simulink library "lib_Convection_LamCircTurbAnnulus"  (R2015a)
settings: Solver=ode45  StartTime=0.0  StopTime=10.0  RelTol=1e-3
settings Model: Creator=jlkratz  LastModifiedBy=jlkratz

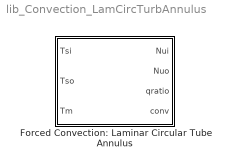
== system lib_Convection_LamCircTurbAnnulus ==
  Forced Convection: Laminar Circular Tube Annulus : Subsystem  mask(TSAT: Forced Convection: Laminar Circular Tube Annulus){Scenario_M=Both surfaces maintain a uniform heat flux, DioDo_M=[0.01 0.5], BN_M=double(gcb)}
      mask prompts: Scenario_M "Scenario_M - Heat transfer scenario"; DioDo_M "DioDo_M - Ratio of inner tube diamter to outer tube diameter (Di/Do) - value(s) shoud be between 0 and 1, if they are not they will be truncated to this range."; BN_M "BN_M - Block Name"
      mask help:
      | This block provides the Nusselt number for fully developed laminar flow within a circular annulus tube. There are two options:
      |
      | (1) one side is insulated and the other has a constant temperature
      | (2) uniform heat flux is maintained at both surfaces
      |
      | The block outputs are the Nusselt numbers associated with the inner and outer surfaces. In case (2) the solutions involves an iterative solver whose solution (the ratio of heat flux's qi/qo) and a parameter indicating convergence of the solution is output. This case also requires additional inputs which include the temperature of both surfaces and the mean temperature of the fluid. Note that the hydraulic diameter, Do - Di in this case, should be used to calculate the convective heat transfer coefficient using the Nusselt numbers from this block.
      |
      | For turbulent flows a circular tube correlation, such as the Dittus-Boelter equation, can be used to get a first approximation of the Nusselt number for both surfaces assuming they are equal and the hydraulic diameter should be used. For more information about this block see the block help menu.
      mask init:
      | %Setup Inputs ------------------------------------------------------------%
      | 
      | % Inport Numbers
      | n = 1; %first inport number
      | 
      | % Inner Surface Temperature (Tsi)
      | if Scenario_M == 2
      |     if strcmp(get_param([gcb '/Tsi'],'BlockType'),'Constant')
      |         MSK_ReplaceBlock_TMATS([gcb '/Tsi'],'built-in/Inport');
      |     end
      |     set_param([gcb '/Tsi'],'Port',num2str(n));
      |     n = n + 1;
      | else
      |     if strcmp(get_param([gcb '/Tsi'],'BlockType'),'Inport')
      |         MSK_ReplaceBlock_TMATS([gcb '/Tsi'],'built-in/Constant');
      |         set_param([gcb '/Tsi'],'Value','700');
      |     end
      | end
      | 
      | % Outer Surface Temperature (Tso)
      | if Scenario_M == 2
      |     if strcmp(get_param([gcb '/Tso'],'BlockType'),'Constant')
      |         MSK_ReplaceBlock_TMATS([gcb '/Tso'],'built-in/Inport');
      |     end
      |     set_param([gcb '/Tso'],'Port',num2str(n));
      |     n = n + 1;
      | else
      |     if strcmp(get_param([gcb '/Tso'],'BlockType'),'Inport')
      |         MSK_ReplaceBlock_TMATS([gcb '/Tso'],'built-in/Constant');
      |         set_param([gcb '/Tso'],'Value','500');
      |     end
      | end
      | 
      | % Mean Fluid Temperature (Tm)
      | if Scenario_M == 2
      |     if strcmp(get_param([gcb '/Tm'],'BlockType'),'Constant')
      |         MSK_ReplaceBlock_TMATS([gcb '/Tm'],'built-in/Inport');
      |     end
      |     set_param([gcb '/Tm'],'Port',num2str(n));
      |     n = n + 1;
      | else
      |     if strcmp(get_param([gcb '/Tm'],'BlockType'),'Inport')
      |         MSK_ReplaceBlock_TMATS([gcb '/Tm'],'built-in/Constant');
      |         set_param([gcb '/Tm'],'Value','400');
      |     end
      | end
      | 
      | %Setup Outputs -----------------------------------------------------------%
      | 
      | % Outport Numbers
      | n = 3; %first inport number
      | 
      | % Uniform heat flux ratio (qratio)
      | if Scenario_M == 2
      |     if strcmp(get_param([gcb '/qratio'],'BlockType'),'Terminator')
      |         MSK_ReplaceBlock_TMATS([gcb '/qratio'],'built-in/Outport');
      |     end
      |     set_param([gcb '/qratio'],'Port',num2str(n));
      |     n = n + 1;
      | else
      |     if strcmp(get_param([gcb '/qratio'],'BlockType'),'Outport')
      |         MSK_ReplaceBlock_TMATS([gcb '/qratio'],'built-in/Terminator');
      |         %set_param([gcb '/qratio'],'Value','1');
      |     end
      | end
      | 
      | % Convergence varialbe for qratio solution (conv)
      | if Scenario_M == 2
      |     if strcmp(get_param([gcb '/conv'],'BlockType'),'Terminator')
      |         MSK_ReplaceBlock_TMATS([gcb '/conv'],'built-in/Outport');
      |     end
      |     set_param([gcb '/conv'],'Port',num2str(n));
      |     n = n + 1;
      | else
      |     if strcmp(get_param([gcb '/conv'],'BlockType'),'Outport')
      |         MSK_ReplaceBlock_TMATS([gcb '/conv'],'built-in/Terminator');
      |         %set_param([gcb '/conv'],'Value','1');
      |     end
      | end
      mask Help: web(which('Convection_TSAT_LamCircTubeAnnulus.html'),'-helpbrowser')
      mask TypeOptions Scenario_M: One surface is insulated and the other is at a constant temperature | Both surfaces maintain a uniform heat flux

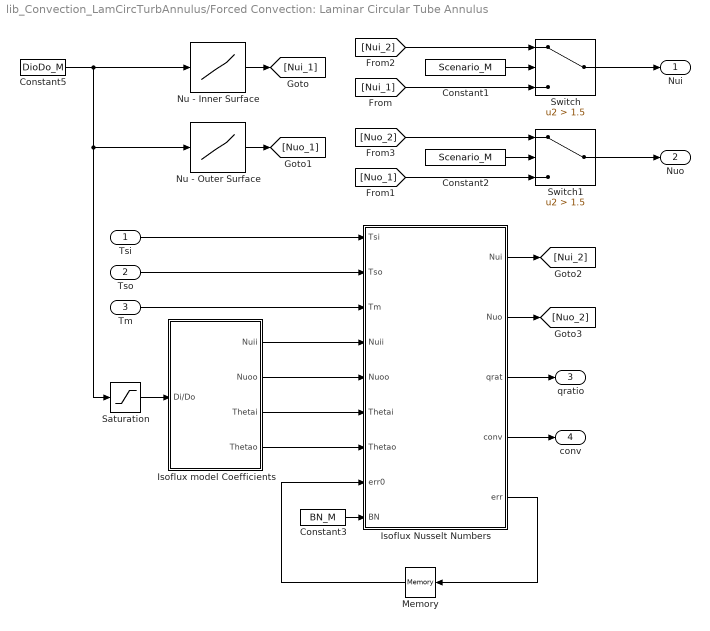
== system lib_Convection_LamCircTurbAnnulus/Forced Convection: Laminar Circular Tube Annulus ==
  Tsi : Inport
  Tso : Inport  Port=2
  Tm : Inport  Port=3
  Constant1 : Constant  Value=Scenario_M
  Constant2 : Constant  Value=Scenario_M
  Constant3 : Constant  Value=BN_M
  Constant5 : Constant  Value=DioDo_M
  Isoflux Nusselt Numbers : MATLAB Function  TreatAsAtomicUnit=on
  "Isoflux model Coefficients " : Subsystem
  Memory : Memory  X0=zeros(1,10)
  Nu - Inner Surface : Lookup_n-D  NumberOfTableDimensions=1  BreakpointsForDimension1=[0 0.05 0.1 0.25 0.5 1]  Table=[17.46 17.46 11.56 7.37 5.74 4.86]  InternalRulePriority=Speed  RndMeth=Simplest  InputSameDT=on
  Nu - Outer Surface : Lookup_n-D  NumberOfTableDimensions=1  BreakpointsForDimension1=[0 0.05 0.1 0.25 0.5 1]  Table=[3.66 4.06 4.11 4.23 4.43 4.86]  InternalRulePriority=Speed  RndMeth=Simplest  InputSameDT=on
  Saturation : Saturate  UpperLimit=1  LowerLimit=0.000001
  Switch : Switch  Criteria=u2 > Threshold  Threshold=1.5
  Switch1 : Switch  Criteria=u2 > Threshold  Threshold=1.5
  Nui : Outport
  Nuo : Outport  Port=2
  qratio : Outport  Port=3
  conv : Outport  Port=4
  wires:
  Saturation/1 -> "Isoflux model Coefficients "/1(Di/Do)
  Memory/1 -> Isoflux Nusselt Numbers/8(err0)
  Constant3/1 -> Isoflux Nusselt Numbers/9(BN)
  Isoflux Nusselt Numbers/5(err) -> Memory/1
  Switch1/1 -> Nuo/1
  Switch/1 -> Nui/1
  Constant2/1 -> Switch1/2
  [Nuo_1] -> Switch1/3
  [Nuo_2] -> Switch1/1
  [Nui_1] -> Switch/3
  [Nui_2] -> Switch/1
  Constant1/1 -> Switch/2
  "Isoflux model Coefficients "/4(Thetao) -> Isoflux Nusselt Numbers/7(Thetao)
  "Isoflux model Coefficients "/3(Thetai) -> Isoflux Nusselt Numbers/6(Thetai)
  "Isoflux model Coefficients "/2(Nuoo) -> Isoflux Nusselt Numbers/5(Nuoo)
  "Isoflux model Coefficients "/1(Nuii) -> Isoflux Nusselt Numbers/4(Nuii)
  Constant5/1 -> Nu - Outer Surface/1, Saturation/1, Nu - Inner Surface/1
  Tm/1 -> Isoflux Nusselt Numbers/3(Tm)
  Tso/1 -> Isoflux Nusselt Numbers/2(Tso)
  Tsi/1 -> Isoflux Nusselt Numbers/1(Tsi)
  Isoflux Nusselt Numbers/4(conv) -> conv/1
  Isoflux Nusselt Numbers/3(qrat) -> qratio/1
  Isoflux Nusselt Numbers/2(Nuo) -> [Nuo_2]
  Isoflux Nusselt Numbers/1(Nui) -> [Nui_2]
  Nu - Outer Surface/1 -> [Nuo_1]
  Nu - Inner Surface/1 -> [Nui_1]

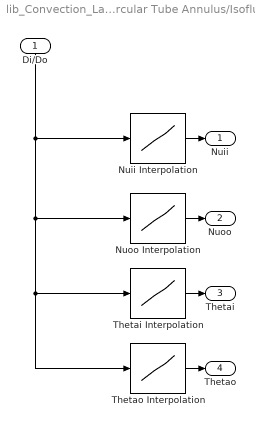
== system lib_Convection_LamCircTurbAnnulus/Forced Convection: Laminar Circular Tube Annulus/Isoflux model Coefficients  ==
  Di/Do : Inport
  Nuii Interpolation : Lookup_n-D  NumberOfTableDimensions=1  BreakpointsForDimension1=[0 0.000001 0.05 0.1 0.2 0.4 0.6 0.8 1]  Table=[0 17.81 17.81 11.91 8.499 6.583 5.912 5.58 5.385]  InternalRulePriority=Speed  RndMeth=Simplest  InputSameDT=on
  Nuoo Interpolation : Lookup_n-D  NumberOfTableDimensions=1  BreakpointsForDimension1=[0 0.05 0.1 0.2 0.4 0.6 0.8 1]  Table=[4.364 4.792 4.834 4.833 4.979 5.099 5.24 5.385]  InternalRulePriority=Speed  RndMeth=Simplest  InputSameDT=on
  Thetai Interpolation : Lookup_n-D  NumberOfTableDimensions=1  BreakpointsForDimension1=[0 0.000001 0.05 0.1 0.2 0.4 0.6 0.8 1]  Table=[0 2.18 2.18 1.383 0.905 0.603 0.473 0.401 0.346]  InternalRulePriority=Speed  RndMeth=Simplest  InputSameDT=on
  Thetao Interpolation : Lookup_n-D  NumberOfTableDimensions=1  BreakpointsForDimension1=[0 0.05 0.1 0.2 0.4 0.6 0.8 1]  Table=[0 0.0294 0.0562 0.1041 0.1823 0.2455 0.299 0.346]  InternalRulePriority=Speed  RndMeth=Simplest  InputSameDT=on
  Nuii : Outport
  Nuoo : Outport  Port=2
  Thetai : Outport  Port=3
  Thetao : Outport  Port=4
  wires:
  Nuii Interpolation/1 -> Nuii/1
  Nuoo Interpolation/1 -> Nuoo/1
  Thetao Interpolation/1 -> Thetao/1
  Di/Do/1 -> Nuii Interpolation/1, Nuoo Interpolation/1, Thetai Interpolation/1, Thetao Interpolation/1
  Thetai Interpolation/1 -> Thetai/1

== matlab function lib_Convection_LamCircTurbAnnulus/Forced Convection: Laminar Circular Tube Annulus/Isoflux Nusselt Numbers ==
  data: Nui output; Nuo output; qrat output; conv output; Tsi input; Tso input; Tm input; Nuii input; Nuoo input; Thetai input; Thetao input; err0 input; BN input; err output
function [Nui,Nuo,qrat,conv,err] = IsofluxSurfaces(Tsi, Tso, Tm, Nuii, Nuoo, Thetai, Thetao, err0, BN)
%#codegen

%Warning/Error Check
err = err0;
errNum = 1;
%Tsi is a 1-D array?
if min(size(Tsi)) ~= 1 && err0(errNum) ~= 1
    fprintf('warning in %s: Tsi must be a scalar or 1-D array\n',char(BN));
    err(errNum) = 1;
end
errNum = errNum + 1;
%Tso is a 1-D array?
if min(size(Tso)) ~= 1 && err0(errNum) ~= 1
    fprintf('warning in %s: Tso must be a scalar or 1-D array\n',char(BN));
    err(errNum) = 1;
end
errNum = errNum + 1;
%Tm is a 1-D array?
if min(size(Tm)) ~= 1 && err0(errNum) ~= 1
    fprintf('warning in %s: Tm must be a scalar or 1-D array\n',char(BN));
    err(errNum) = 1;
end
errNum = errNum + 1;
%Tsi, Tso, Tm, and DioDo_m (Nuii, Nuoo, Thetai, and Thetao) are the same size?
if (length(Tsi) ~= length(Tso) || length(Tsi) ~= length(Tm) || length(Tsi) ~= length(Nuii)) && err0(errNum) ~= 1
    fprintf('warning in %s: Tsi, Tso, Tm and DioDo_M must have the same number of elements\n',char(BN));
    err(errNum) = 1;
end
errNum = errNum + 1;
%Tsi has all real elements?
if min(isreal(Tsi)) < 1 && err0(errNum) ~= 1
    fprintf('warning in %s: Tsi must have all real elements\n',char(BN));
    err(errNum) = 1;
end
errNum = errNum + 1;
%Tso has all real elements?
if min(isreal(Tso)) < 1 && err0(errNum) ~= 1
    fprintf('warning in %s: Tso must have all real elements\n',char(BN));
    err(errNum) = 1;
end
errNum = errNum + 1;
%Tm has all real elements?
if min(isreal(Tm)) < 1 && err0(errNum) ~= 1
    fprintf('warning in %s: Tm must have all real elements\n',char(BN));
    err(errNum) = 1;
end
errNum = errNum + 1;
%Tsi has all finite elements?
if (max(isnan(Tsi)) > 0 || max(isinf(Tsi)) > 0) && err0(errNum) ~= 1
    fprintf('warning in %s: Tsi must have all finite elements\n',char(BN));
    err(errNum) = 1;
end
errNum = errNum + 1;
%Tso has all finite elements?
if (max(isnan(Tso)) > 0 || max(isinf(Tso)) > 0) && err0(errNum) ~= 1
    fprintf('warning in %s: Tso must have all finite elements\n',char(BN));
    err(errNum) = 1;
end
%Tm has all finite elements?
if (max(isnan(Tm)) > 0 || max(isinf(Tm)) > 0) && err0(errNum) ~= 1
    fprintf('warning in %s: Tm must have all finite elements\n',char(BN));
    err(errNum) = 1;
end

%Max number of iterations
imax = 1000;

%Initialize outputs
Nui = zeros(1,length(Tsi));
Nuo = zeros(1,length(Tsi));
qrat = zeros(1,length(Tsi));
conv = zeros(1,length(Tsi));

for j = 1:length(Tsi)

    %vector of the variable being solve for
    dT1 = Tsi(j) - Tm(j);
    dT2 = Tso(j) - Tm(j);
    a = abs(15*dT1/dT2);
    n = 100;
    qrat_vect = linspace(-a,a,n);

    %find the appropriate root
    if sign(Tsi(j)-Tm(j)) == sign(Tso(j)-Tm(j))
        Fend = qrat_vect(end) - (Nuii(j)/(1 - (1/qrat_vect(end))*Thetai(j))) * ((1 - qrat_vect(end)*Thetao(j))/Nuoo(j)) * (Tsi(j) - Tm(j))/(Tso(j) - Tm(j));
        signFend = sign(Fend);
        i = length(qrat_vect)-1;
        cnt = 0;
        Fi = qrat_vect(i) - (Nuii(j)/(1 - (1/qrat_vect(i))*Thetai(j))) * ((1 - qrat_vect(i)*Thetao(j))/Nuoo(j)) * (Tsi(j) - Tm(j))/(Tso(j) - Tm(j));
        while sign(Fi) == signFend && cnt < imax
            i = i - 1;
            cnt = cnt + 1;
            Fi = qrat_vect(i) - (Nuii(j)/(1 - (1/qrat_vect(i))*Thetai(j))) * ((1 - qrat_vect(i)*Thetao(j))/Nuoo(j)) * (Tsi(j) - Tm(j))/(Tso(j) - Tm(j));
        end
        conv(j) = 1;
        if cnt == imax
            conv(j) = 0;
        end
        qrat_a = qrat_vect(i);
        Fa = qrat_a - (Nuii(j)/(1 - (1/qrat_a)*Thetai(j))) * ((1 - qrat_a*Thetao(j))/Nuoo(j)) * (Tsi(j) - Tm(j))/(Tso(j) - Tm(j));
        qrat_b = qrat_vect(i+1);
        Fb = qrat_b - (Nuii(j)/(1 - (1/qrat_b)*Thetai(j))) * ((1 - qrat_b*Thetao(j))/Nuoo(j)) * (Tsi(j) - Tm(j))/(Tso(j) - Tm(j));
    else
        F1 = qrat_vect(1) - (Nuii(j)/(1 - (1/qrat_vect(1))*Thetai(j))) * ((1 - qrat_vect(1)*Thetao(j))/Nuoo(j)) * (Tsi(j) - Tm(j))/(Tso(j) - Tm(j));
        signF1 = sign(F1);
        i = 2;
        cnt = 0;
        Fi = qrat_vect(i) - (Nuii(j)/(1 - (1/qrat_vect(i))*Thetai(j))) * ((1 - qrat_vect(i)*Thetao(j))/Nuoo(j)) * (Tsi(j) - Tm(j))/(Tso(j) - Tm(j));
        while sign(Fi) == signF1 && cnt < imax
            i = i + 1;
            cnt = cnt + 1;
            Fi = qrat_vect(i) - (Nuii(j)/(1 - (1/qrat_vect(i))*Thetai(j))) * ((1 - qrat_vect(i)*Thetao(j))/Nuoo(j)) * (Tsi(j) - Tm(j))/(Tso(j) - Tm(j));
        end
        conv(j) = 1;
        if cnt == imax
            conv(j) = 0;
        end
        qrat_a = qrat_vect(i-1);
        Fa = qrat_a - (Nuii(j)/(1 - (1/qrat_a)*Thetai(j))) * ((1 - qrat_a*Thetao(j))/Nuoo(j)) * (Tsi(j) - Tm(j))/(Tso(j) - Tm(j));
        qrat_b = qrat_vect(i);
        Fb = qrat_b - (Nuii(j)/(1 - (1/qrat_b)*Thetai(j))) * ((1 - qrat_b*Thetao(j))/Nuoo(j)) * (Tsi(j) - Tm(j))/(Tso(j) - Tm(j));
    end
    qrat(j) = (0-Fa)/(Fb-Fa) * (qrat_b-qrat_a) + qrat_a;

    %Calculate the Nusselt Numbers
    Nui(j) = Nuii(j)/(1 - (1/qrat(j))*Thetai(j));
    Nuo(j) = Nuoo(j)/(1 - qrat(j)*Thetao(j));

end

end
